simulink library "battery_model_lib"  (R2022b)
settings: Solver=VariableStepAuto  StartTime=0.0  StopTime=10.0  RelTol=1e-3
settings Model: Creator=dr_pa  LastModifiedBy=dr_pa

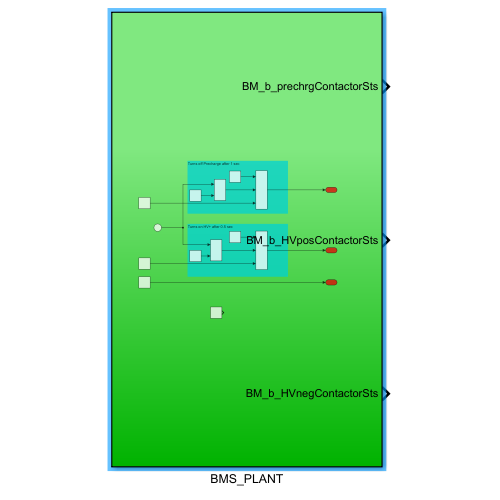
[thumbnail: Simulink's stored preview of the top-level diagram]
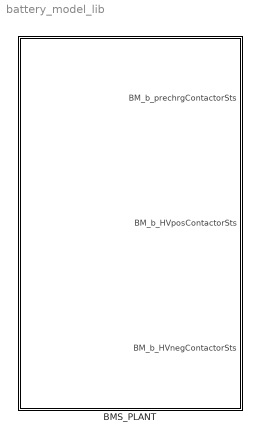
== system battery_model_lib ==
  BMS_PLANT : Subsystem

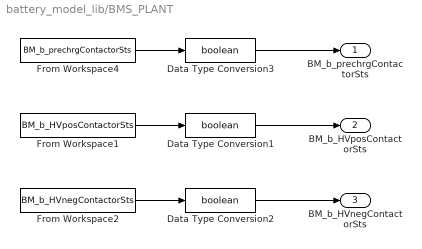
== system battery_model_lib/BMS_PLANT ==
  Data Type Conversion1 : DataTypeConversion  OutDataTypeStr=boolean  SaturateOnIntegerOverflow=off  RndMeth=Floor
  Data Type Conversion2 : DataTypeConversion  OutDataTypeStr=boolean  SaturateOnIntegerOverflow=off  RndMeth=Floor
  Data Type Conversion3 : DataTypeConversion  OutDataTypeStr=boolean  SaturateOnIntegerOverflow=off  RndMeth=Floor
  From Workspace1 : FromWorkspace  VariableName=BM_b_HVposContactorSts
  From Workspace2 : FromWorkspace  VariableName=BM_b_HVnegContactorSts
  From Workspace4 : FromWorkspace  VariableName=BM_b_prechrgContactorSts
  BM_b_prechrgContactorSts : Outport
  BM_b_HVposContactorSts : Outport  Port=2
  BM_b_HVnegContactorSts : Outport  Port=3
  wires:
  From Workspace4/1 -> Data Type Conversion3/1
  Data Type Conversion3/1 -> BM_b_prechrgContactorSts/1
  From Workspace1/1 -> Data Type Conversion1/1
  Data Type Conversion1/1 -> BM_b_HVposContactorSts/1
  Data Type Conversion2/1 -> BM_b_HVnegContactorSts/1
  From Workspace2/1 -> Data Type Conversion2/1
